simulink model "pp_integral_action_sym"  (R2023b)
settings: Solver=VariableStepAuto  StartTime=0.0  StopTime=15  RelTol=1e-3
values from neighbouring files (symbols this model uses):
  A = [-p1-x2_eq -x1_eq; 0 -p2]    [WP2.m]    (also in lqr.m)
  B = [0; p3]    [WP2.m]    (also in lqr.m)
  C = [1 0]    [WP2.m]    (also in lqr.m)
  K = place(Atilde, [B; 0], [-10 -15 -20])    [WP2.m]    (also in lqr.m = lqr(sys, Qx, Qu))
settings Model: Creator=kiraa  LastModifiedBy=kiraa

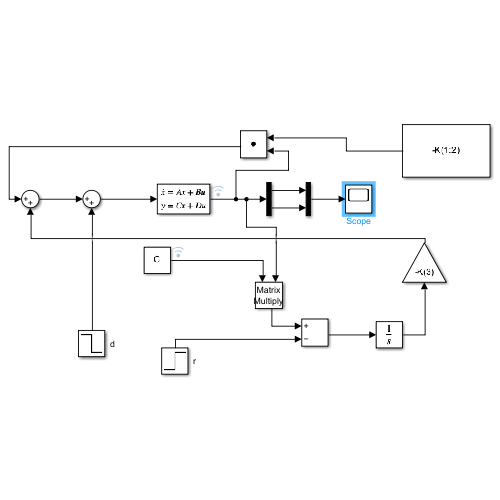
[thumbnail: Simulink's stored preview of the top-level diagram]
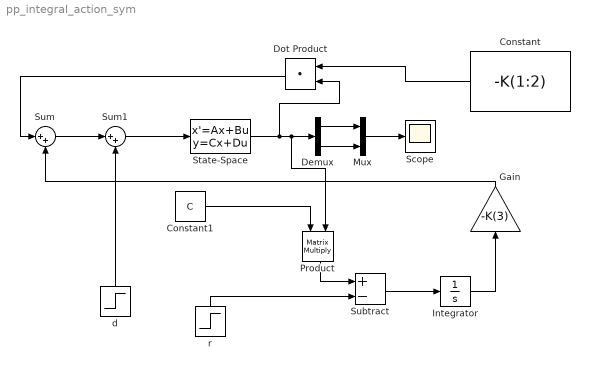
== system pp_integral_action_sym ==
  Constant : Constant  Value=-K(1:2)
  Constant1 : Constant  Value=C  VectorParams1D=off
  Demux : Demux  Outputs=2
  Dot Product : DotProduct  InputSameDT=off  OutDataTypeStr=Inherit: Inherit via internal rule
  Gain : Gain  Gain=-K(3)
  Integrator : Integrator
  Mux : Mux  Inputs=2
  Product : Product  Multiplication=Matrix(*)
  Scope : Scope
  State-Space : StateSpace  A=A  B=B  C=eye(2)  D=[0; 0]  InitialCondition=[0 0]  ParameterTunability=Unconstrained
  Subtract : Sum  Inputs=+-
  Sum : Sum  Inputs=|++
  Sum1 : Sum  Inputs=|++
  d : Step  Time=8  After=-2  SampleTime=0
  r : Step  After=5  SampleTime=0
  wires:
  Dot Product/1 -> Sum/1
  Sum/1 -> Sum1/1
  Demux/1 -> Mux/1
  Demux/2 -> Mux/2
  Mux/1 -> Scope/1
  r/1 -> Subtract/2
  Subtract/1 -> Integrator/1
  Integrator/1 -> Gain/1
  Gain/1 -> Sum/2
  Constant/1 -> Dot Product/1
  Sum1/1 -> State-Space/1
  d/1 -> Sum1/2
  Constant1/1 -> Product/1
  State-Space/1 -> Dot Product/2, Product/2, Demux/1
  Product/1 -> Subtract/1
